simulink model "sfcndemo_sfun_fcncall"  (Simulink 6.0)
settings: Solver=FixedStepDiscrete  SolverMode=SingleTasking  StartTime=0.0  StopTime=1  FixedStep=.1  RelTol=1e-3  AbsTol=1e-6
settings Model: Creator=The MathWorks Inc.  LastModifiedBy=batserve  ExtModeTrigMode=oneshot  ExtModeArmWhenConnect=off  ExtModeAutoUpdateStatusClock=off
settings DataIOCC: LimitDataPoints=off  SignalLoggingName=sigsOut
settings OptimizationCC: BooleanDataType=off
settings DebuggingCC: CheckExecutionContextPreStartOutputMsg=on  CheckExecutionContextRuntimeOutputMsg=on  SolverPrmCheckMsg=none  InheritedTsInSrcMsg=none
settings HardwareCC: TargetUnknown=on

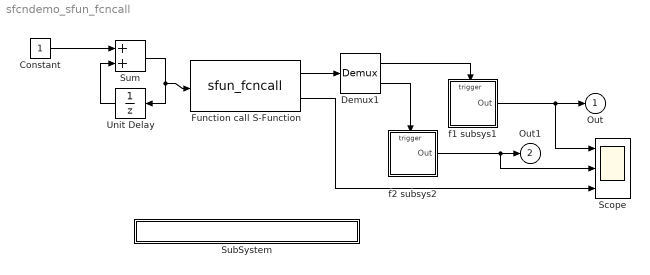
== system sfcndemo_sfun_fcncall ==
  Constant : Constant
  Demux1 : Demux  Outputs=2
  Function call S-Function : S-Function  FunctionName=sfun_fcncall
      mask Type: S-function: sfun_fcncall
      mask Description: This is a S-function block which is configure to execute "function-call" subsystems on the 1st and 3rd output element of the output port. Note when performing function-calls, these can only be done through the 1st output port.
  Scope : Scope  NumInputPorts=3
      settings: TimeRange=1  YMin=0~0~0  YMax=1~10~10
  SubSystem : Subsystem  PropExecContextAcrossSSBoundary=on
      settings: OpenFcn=edit(fullfile(matlabroot,'simulink','src','sfun_fcncall.c'))
      mask Display: disp('matlabroot\simulink\src\sfun_fcncall.c');
  Sum : Sum  SaturateOnIntegerOverflow=on  InputSameDT=on
  Unit Delay : UnitDelay  Orientation=left  SampleTime=.1
  f1 subsys1 : Subsystem  TreatAsAtomicUnit=on  PropExecContextAcrossSSBoundary=on
  f2 subsys2 : Subsystem  TreatAsAtomicUnit=on  PropExecContextAcrossSSBoundary=on
  Out : Outport  InitialOutput=0
  Out1 : Outport  Port=2  InitialOutput=0
  wires:
  Sum/1 -> Unit Delay/1, Function call S-Function/1
  Demux1/2 -> f2 subsys2/Trigger
  Function call S-Function/1 -> Demux1/1
  Constant/1 -> Sum/1
  Unit Delay/1 -> Sum/2
  f1 subsys1/1(Out) -> Out/1, Scope/1
  Demux1/1 -> f1 subsys1/Trigger
  Function call S-Function/2 -> Scope/3
  f2 subsys2/1(Out) -> Out1/1, Scope/2

== system sfcndemo_sfun_fcncall/SubSystem ==

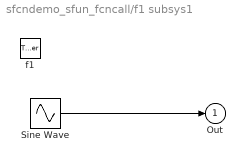
== system sfcndemo_sfun_fcncall/f1 subsys1 ==
  f1 : TriggerPort  TriggerType=function-call
  Sine Wave : Sin
  Out : Outport  InitialOutput=0
  wires:
  Sine Wave/1 -> Out/1

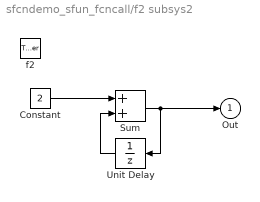
== system sfcndemo_sfun_fcncall/f2 subsys2 ==
  f2 : TriggerPort  TriggerType=function-call
  Constant : Constant  Value=2
  Sum : Sum  SaturateOnIntegerOverflow=on  InputSameDT=on
  Unit Delay : UnitDelay  Orientation=left  SampleTime=-1
  Out : Outport  InitialOutput=0
  wires:
  Constant/1 -> Sum/1
  Unit Delay/1 -> Sum/2
  Sum/1 -> Unit Delay/1, Out/1
